simulink model "L8_PT"  (R2016a)
settings: Solver=VariableStepAuto  StartTime=0.0  StopTime=10.0  RelTol=1e-3
libraries: dsparch4 x1, commsynccomp2 x1
settings Model: Creator=AIUB  LastModifiedBy=AIUB

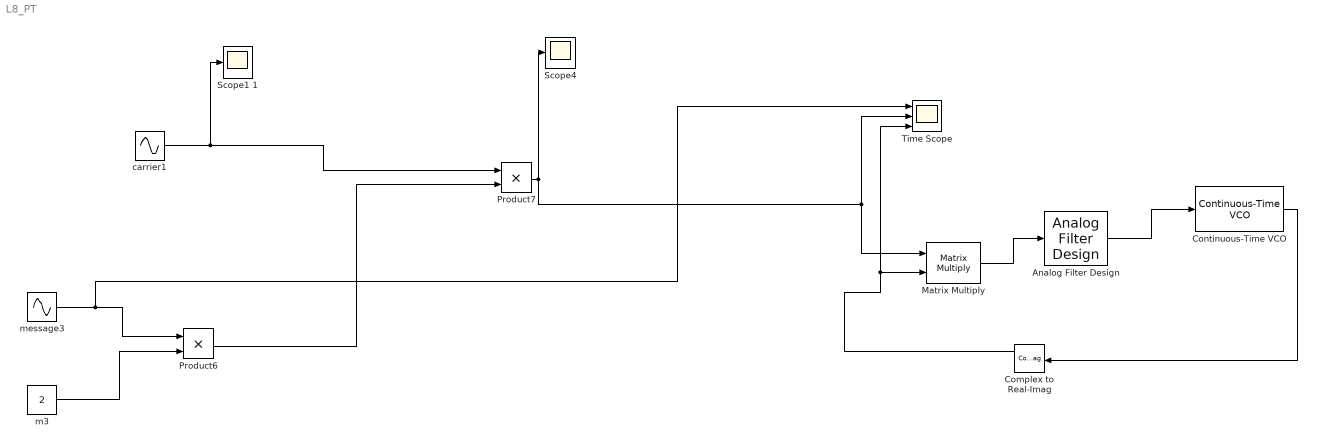
== system L8_PT ==
  " carrier1" : Sin  Frequency=2*pi*50  SampleTime=1/5000
  " message3" : Sin  SineType=Sample based  Amplitude=2  Frequency=2*pi*10+pi/3  SampleTime=1/5000
  Analog Filter Design : dsparch4/Analog Filter Design  method=Butterworth  filttype=Lowpass  N=10  Wlo=2*pi*10  Whi=80  Rp=2  Rs=40
  Complex to Real-Imag : ComplexToRealImag
  Continuous-Time VCO : commsynccomp2/Continuous-Time VCO  Ac=1  Fc=10  Kc=50  Ph=0
  Matrix Multiply : Product  Multiplication=Matrix(*)
  Product6 : Product
  Product7 : Product
  Scope1 1 : Scope
  Scope4 : Scope
  Time Scope : Scope  NumInputPorts=3
  m3 : Constant  Value=2
  wires:
  Product7/1 -> Matrix Multiply/1, Time Scope/2, Scope4/1
  Continuous-Time VCO/1 -> Complex to Real-Imag/1
  Complex to Real-Imag/1 -> Time Scope/3, Matrix Multiply/2
  Matrix Multiply/1 -> Analog Filter Design/1
  Analog Filter Design/1 -> Continuous-Time VCO/1
  " message3"/1 -> Time Scope/1, Product6/1
  " carrier1"/1 -> Product7/1, Scope1 1/1
  Product6/1 -> Product7/2
  m3/1 -> Product6/2
